simulink model "data_collection"  (R2024a)
settings: Solver=FixedStepAuto  StartTime=0.0  StopTime=inf  FixedStep=0.01  RelTol=1e-3
values from neighbouring files (symbols this model uses):
  omega_max = Simulink.Parameter(425.47)    [katech_automation.m]
  wind_type_toggle = 2    [katech_automation.m]    (also in katech_automation_HILS.m)
  window_size_ = Simulink.Parameter(100)    [katech_automation.m]    (also in katech_automation_HILS.m)
undefined symbols (not defined in the file or in its folder): rad, s, X, Y, Z
libraries: robotlib x28, simulink x14, aerolibconvert2 x2, sharedtransform x1, simulink_extras x1, eeGeneralControl x1
(part 2 of 2)

== matlab function data_collection/MATLAB Function11 ==
  data: wind_x_flag input; wind_y_flag input; u input; y output; toggle_swtich output
function [y, toggle_swtich] = fcn(wind_x_flag, wind_y_flag, u)
    coder.extrinsic('assignin'); % MATLAB 함수 사용을 알림


    % 이전 값을 저장할 persistent 변수 선언
    persistent prev_u;
    persistent toggle_state;
    persistent prev_flag;

    if isempty(prev_u)
        prev_u = -inf; % 초기 값 설정
    end

    if isempty(toggle_state)
        toggle_state = false; % 초기 토글 상태를 논리형으로 설정
    end

    if isempty(prev_flag)
        prev_flag    = false;
    end

    
    % 현재 플래그 레벨
    curr_flag = wind_x_flag || wind_y_flag;

    % 상승엣지 검출: 이전=0 & 현재=1
    if curr_flag && ~prev_flag
        toggle_state = ~toggle_state;
    end

    prev_flag = curr_flag;    % 엣지 검출을 위한 상태 갱신

    % 현재 토글 상태를 int32 형으로 변환하여 할당
    toggle_swtich = int32(toggle_state);
    % 현재 토글 상태를 출력
    % fprintf('toggle_state = %d \n', toggle_swtich);

    if toggle_state
        % 현재 값이 이전 값보다 큰지 확인
        if u > prev_u
            
            prev_u = u; % 이전 값을 현재 값으로 업데이트
            y = u; % 현재 값을 출력
        else
            y = prev_u; % 이전 값을 출력
        end
        assignin('base', 'max_z_error', y); % y 값을 MATLAB 기본 워크스페이스의 xy_error에 저장
    else
        % 토글 상태가 0일 때
        prev_u = 0;
        y = 0;
    end
end




    % if x_change || y_change
    % 
    %     % 현재 값이 이전 값보다 큰지 확인
    %     if u > prev_u
    %         assignin('base', 'xy_error', u);  % u 값을 MATLAB  워크스페이스(base는 MATLAB의 기본 워크스페이스를 의미)의 xy_error에 저장
    %         prev_u = u; % 이전 값을 현재 값으로 업데이트
    %         y = u; % 현재 값을 출력
    %     else
    %         y = prev_u; % 이전 값을 출력
    %     end
    % else
    %     assignin('base', 'xy_error', u);
    %     y = 0;
    % end

== matlab function data_collection/MATLAB Function12 ==
  data: endstep_xyz_error input; y output
function y = fcn(endstep_xyz_error)

% z_error 값을 기본 워크스페이스에 저장
assignin('base', 'endstep_xyz_error', endstep_xyz_error);

% 저장된 값을 반환
y = endstep_xyz_error;

end

== matlab function data_collection/MATLAB Function13 ==
  data: wind_toggle input; x_flag output; a1 input; a2 input; a3 input; a4 input; y_flag output
function [x_flag,y_flag] = fcn(wind_toggle,a1,a2,a3,a4)

% If wind_toggle is 
% 1 : Gust
% 2 : Normal Distribution
if wind_toggle == 1
    x_flag = a1;
    y_flag = a2;
else
    x_flag = a3;
    y_flag = a4;
end

end

== matlab function data_collection/MATLAB Function14 ==
  data: wind_x_flag input; wind_y_flag input; u input; y output; toggle_swtich output
function [y, toggle_swtich] = fcn(wind_x_flag, wind_y_flag, u)
    coder.extrinsic('assignin'); % MATLAB 함수 사용을 알림


    % 이전 값을 저장할 persistent 변수 선언
    persistent prev_u;
    persistent toggle_state;
    persistent prev_flag;

    if isempty(prev_u)
        prev_u = -inf; % 초기 값 설정
    end

    if isempty(toggle_state)
        toggle_state = false; % 초기 토글 상태를 논리형으로 설정
    end

    if isempty(prev_flag)
        prev_flag    = false;
    end

    
    % 현재 플래그 레벨
    curr_flag = wind_x_flag || wind_y_flag;

    % 상승엣지 검출: 이전=0 & 현재=1
    if curr_flag && ~prev_flag
        toggle_state = ~toggle_state;
    end

    prev_flag = curr_flag;    % 엣지 검출을 위한 상태 갱신

    % 현재 토글 상태를 int32 형으로 변환하여 할당
    toggle_swtich = int32(toggle_state);
    % 현재 토글 상태를 출력
    % fprintf('toggle_state = %d \n', toggle_swtich);

    if toggle_state
        % 현재 값이 이전 값보다 큰지 확인
        if u > prev_u
            
            prev_u = u; % 이전 값을 현재 값으로 업데이트
            y = u; % 현재 값을 출력
        else
            y = prev_u; % 이전 값을 출력
        end
        assignin('base', 'max_x_error', y); % y 값을 MATLAB 기본 워크스페이스의 xy_error에 저장
    else
        % 토글 상태가 0일 때
        prev_u = 0;
        y = 0;
    end
end




    % if x_change || y_change
    % 
    %     % 현재 값이 이전 값보다 큰지 확인
    %     if u > prev_u
    %         assignin('base', 'xy_error', u);  % u 값을 MATLAB  워크스페이스(base는 MATLAB의 기본 워크스페이스를 의미)의 xy_error에 저장
    %         prev_u = u; % 이전 값을 현재 값으로 업데이트
    %         y = u; % 현재 값을 출력
    %     else
    %         y = prev_u; % 이전 값을 출력
    %     end
    % else
    %     assignin('base', 'xy_error', u);
    %     y = 0;
    % end

== matlab function data_collection/Subsystem2/MATLAB Function5 ==
  data: wind_x_flag input; wind_y_flag input; u input; y output; toggle_swtich output
function [y, toggle_swtich] = fcn(wind_x_flag, wind_y_flag, u)
    coder.extrinsic('assignin'); % MATLAB 함수 사용을 알림


    % 이전 값을 저장할 persistent 변수 선언
    persistent prev_u;
    persistent toggle_state;
    persistent prev_flag;

    if isempty(prev_u)
        prev_u = -inf; % 초기 값 설정
    end

    if isempty(toggle_state)
        toggle_state = false; % 초기 토글 상태를 논리형으로 설정
    end

    if isempty(prev_flag)
        prev_flag    = false;
    end

    % 현재 플래그 레벨
    curr_flag = wind_x_flag || wind_y_flag;

    % 상승엣지 검출: 이전=0 & 현재=1
    if curr_flag && ~prev_flag
        toggle_state = ~toggle_state;
    end

    prev_flag = curr_flag;    % 엣지 검출을 위한 상태 갱신

    % 현재 토글 상태를 int32 형으로 변환하여 할당
    toggle_swtich = int32(toggle_state);
    % 현재 토글 상태를 출력
    % fprintf('toggle_state = %d \n', toggle_swtich);

    if toggle_state
        % 현재 값이 이전 값보다 큰지 확인
        if abs(u) > abs(prev_u)
            y = abs(prev_u); % 이전 값을 출력
            
        else
            prev_u = abs(u); % 이전 값을 현재 값으로 업데이트
            y = abs(u); % 현재 값을 출력
        end
        assignin('base', 'min_avg_array_FCM_saturated', y); % y 값을 MATLAB 기본 워크스페이스의 min_FCMW 저장
    else
        % 토글 상태가 0일 때
        prev_u = 1;
        y = 1;
    end
end




    % if x_change || y_change
    % 
    %     % 현재 값이 이전 값보다 큰지 확인
    %     if u > prev_u
    %         assignin('base', 'current_roll', u);  % u 값을 MATLAB  워크스페이스(base는 MATLAB의 기본 워크스페이스를 의미)의 current_roll에 저장
    %         prev_u = u; % 이전 값을 현재 값으로 업데이트
    %         y = u; % 현재 값을 출력
    %     else
    %         y = prev_u; % 이전 값을 출력
    %     end
    % else
    %     assignin('base', 'current_roll', u);
    %     y = 0;
    % end

== matlab function data_collection/MATLAB Function8 ==
  settings: updateMethod=DISCRETE
  data: xyz_error input; avg_array_xyz_error output; window_size_ parameter
function avg_array_xyz_error  = fcn(xyz_error, window_size_)

coder.extrinsic('calculate_xyzerror.m');

% persistent 변수 선언
persistent initialized avg_array_xyz_error_;

% 초기화가 필요할 때만 실행
if isempty(initialized)
    initialized = true; % 초기화 완료 표시
    one_or_zero = 0;
    one_or_zero_ = 0;
    avg_array_xyz_error = 0.0;
    avg_array_xyz_error_ = 0.0;

    disp('initialized. in MATLAB Function8');
    % disp('window_size_ in MATLAB Function8'); disp(window_size_);
end


[one_or_zero_, avg_array_xyz_error_] = calculate_xyzerror(xyz_error,window_size_);

one_or_zero = one_or_zero_;
avg_array_xyz_error = avg_array_xyz_error_;





end

== matlab function data_collection/MATLAB Function15 ==
  data: wind_x_flag input; wind_y_flag input; u input; y output; toggle_swtich output
function [y, toggle_swtich] = fcn(wind_x_flag, wind_y_flag, u)
    coder.extrinsic('assignin'); % MATLAB 함수 사용을 알림


    % 이전 값을 저장할 persistent 변수 선언
    persistent prev_u;
    persistent toggle_state;
    persistent prev_flag;

    if isempty(prev_u)
        prev_u = -inf; % 초기 값 설정
    end

    if isempty(toggle_state)
        toggle_state = false; % 초기 토글 상태를 논리형으로 설정
    end

    if isempty(prev_flag)
        prev_flag    = false;
    end

    
    % 현재 플래그 레벨
    curr_flag = wind_x_flag || wind_y_flag;

    % 상승엣지 검출: 이전=0 & 현재=1
    if curr_flag && ~prev_flag
        toggle_state = ~toggle_state;
    end

    prev_flag = curr_flag;    % 엣지 검출을 위한 상태 갱신

    % 현재 토글 상태를 int32 형으로 변환하여 할당
    toggle_swtich = int32(toggle_state);
    % 현재 토글 상태를 출력
    % fprintf('toggle_state = %d \n', toggle_swtich);

    if toggle_state
        % 현재 값이 이전 값보다 큰지 확인
        if u > prev_u
            
            prev_u = u; % 이전 값을 현재 값으로 업데이트
            y = u; % 현재 값을 출력
        else
            y = prev_u; % 이전 값을 출력
        end
        assignin('base', 'max_avg_xyz_error', y); % y 값을 MATLAB 기본 워크스페이스의 max_avg_xyz_error 에 저장
    else
        % 토글 상태가 0일 때
        prev_u = 0;
        y = 0;
    end
end




    % if x_change || y_change
    % 
    %     % 현재 값이 이전 값보다 큰지 확인
    %     if u > prev_u
    %         assignin('base', 'xy_error', u);  % u 값을 MATLAB  워크스페이스(base는 MATLAB의 기본 워크스페이스를 의미)의 xy_error에 저장
    %         prev_u = u; % 이전 값을 현재 값으로 업데이트
    %         y = u; % 현재 값을 출력
    %     else
    %         y = prev_u; % 이전 값을 출력
    %     end
    % else
    %     assignin('base', 'xy_error', u);
    %     y = 0;
    % end

== matlab function data_collection/MATLAB Function16 ==
  data: u input
function write_pos_err(u)
    assignin('base', 'position_error', u);
end

== matlab function data_collection/Subsystem2/MATLAB Function7 ==
  data: u input
function write_fcmw(u)
    assignin('base', 'FCMW_saturated', u);
end

== matlab function data_collection/MATLAB Function1 ==
  data: wind_x_flag input; wind_y_flag input; u input; y output; toggle_swtich output
function [y, toggle_swtich] = fcn(wind_x_flag, wind_y_flag, u)
    coder.extrinsic('assignin'); % MATLAB 함수 사용을 알림


    % 이전 값을 저장할 persistent 변수 선언
    persistent prev_u;
    persistent toggle_state;
    persistent prev_flag;

    if isempty(prev_u)
        prev_u = -inf; % 초기 값 설정
    end

    if isempty(toggle_state)
        toggle_state = false; % 초기 토글 상태를 논리형으로 설정
    end

    if isempty(prev_flag)
        prev_flag    = false;
    end

    
    % 현재 플래그 레벨
    curr_flag = wind_x_flag || wind_y_flag;

    % 상승엣지 검출: 이전=0 & 현재=1
    if curr_flag && ~prev_flag
        toggle_state = ~toggle_state;
    end

    prev_flag = curr_flag;    % 엣지 검출을 위한 상태 갱신

    % 현재 토글 상태를 int32 형으로 변환하여 할당
    toggle_swtich = int32(toggle_state);
    % 현재 토글 상태를 출력
    % fprintf('toggle_state = %d \n', toggle_swtich);

    if toggle_state
        % 현재 값이 이전 값보다 큰지 확인
        if abs(u) > abs(prev_u)
            
            prev_u = u; % 이전 값을 현재 값으로 업데이트
            y = u; % 현재 값을 출력
        else
            y = prev_u; % 이전 값을 출력
        end
        assignin('base', 'max_roll', y); % y 값을 MATLAB 기본 워크스페이스의 xy_error에 저장
    else
        % 토글 상태가 0일 때
        prev_u = 0;
        y = 0;
    end
end




    % if x_change || y_change
    % 
    %     % 현재 값이 이전 값보다 큰지 확인
    %     if u > prev_u
    %         assignin('base', 'xy_error', u);  % u 값을 MATLAB  워크스페이스(base는 MATLAB의 기본 워크스페이스를 의미)의 xy_error에 저장
    %         prev_u = u; % 이전 값을 현재 값으로 업데이트
    %         y = u; % 현재 값을 출력
    %     else
    %         y = prev_u; % 이전 값을 출력
    %     end
    % else
    %     assignin('base', 'xy_error', u);
    %     y = 0;
    % end

== matlab function data_collection/MATLAB Function ==
  data: wind_x_flag input; wind_y_flag input; u input; y output; toggle_swtich output
function [y, toggle_swtich] = fcn(wind_x_flag, wind_y_flag, u)
    coder.extrinsic('assignin'); % MATLAB 함수 사용을 알림


    % 이전 값을 저장할 persistent 변수 선언
    persistent prev_u;
    persistent toggle_state;
    persistent prev_flag;

    if isempty(prev_u)
        prev_u = -inf; % 초기 값 설정
    end

    if isempty(toggle_state)
        toggle_state = false; % 초기 토글 상태를 논리형으로 설정
    end

    if isempty(prev_flag)
        prev_flag    = false;
    end

    
    % 현재 플래그 레벨
    curr_flag = wind_x_flag || wind_y_flag;

    % 상승엣지 검출: 이전=0 & 현재=1
    if curr_flag && ~prev_flag
        toggle_state = ~toggle_state;
    end

    prev_flag = curr_flag;    % 엣지 검출을 위한 상태 갱신

    % 현재 토글 상태를 int32 형으로 변환하여 할당
    toggle_swtich = int32(toggle_state);
    % 현재 토글 상태를 출력
    % fprintf('toggle_state = %d \n', toggle_swtich);

    if toggle_state
        % 현재 값이 이전 값보다 큰지 확인
        if u > prev_u
            
            prev_u = u; % 이전 값을 현재 값으로 업데이트
            y = u; % 현재 값을 출력
        else
            y = prev_u; % 이전 값을 출력
        end
        assignin('base', 'max_xy_error', y); % y 값을 MATLAB 기본 워크스페이스의 xy_error에 저장
    else
        % 토글 상태가 0일 때
        prev_u = 0;
        y = 0;
    end
end




    % if x_change || y_change
    % 
    %     % 현재 값이 이전 값보다 큰지 확인
    %     if u > prev_u
    %         assignin('base', 'xy_error', u);  % u 값을 MATLAB  워크스페이스(base는 MATLAB의 기본 워크스페이스를 의미)의 xy_error에 저장
    %         prev_u = u; % 이전 값을 현재 값으로 업데이트
    %         y = u; % 현재 값을 출력
    %     else
    %         y = prev_u; % 이전 값을 출력
    %     end
    % else
    %     assignin('base', 'xy_error', u);
    %     y = 0;
    % end

== matlab function data_collection/MATLAB Function2 ==
  data: endstep_z_error input; y output
function y = fcn(endstep_z_error)

% z_error 값을 기본 워크스페이스에 저장
assignin('base', 'endstep_z_error', endstep_z_error);

% 저장된 값을 반환
y = endstep_z_error;

end

== matlab function data_collection/MATLAB Function3 ==
  data: endstep_y_error input; y output
function y = fcn(endstep_y_error)

% z_error 값을 기본 워크스페이스에 저장
assignin('base', 'endstep_y_error', endstep_y_error);

% 저장된 값을 반환
y = endstep_y_error;

end

== matlab function data_collection/MATLAB Function4 ==
  data: endstep_x_error input; y output
function y = fcn(endstep_x_error)

% z_error 값을 기본 워크스페이스에 저장
assignin('base', 'endstep_x_error', endstep_x_error);

% 저장된 값을 반환
y = endstep_x_error;

end

== matlab function data_collection/MATLAB Function5 ==
  data: xy_error input; y output
function y = two_norm(xy_error)
    coder.extrinsic('norm'); % MATLAB 함수 사용을 알림
    
    

    
    % 'y'를 명확히 초기화
    y = 0; 
    
y = norm(xy_error,2);

== matlab function data_collection/MATLAB Function6 ==
  data: wind_x_flag input; wind_y_flag input; u input; y output; toggle_swtich output
function [y, toggle_swtich] = fcn(wind_x_flag, wind_y_flag, u)
    coder.extrinsic('assignin'); % MATLAB 함수 사용을 알림


    % 이전 값을 저장할 persistent 변수 선언
    persistent prev_u;
    persistent toggle_state;
    persistent prev_flag;

    if isempty(prev_u)
        prev_u = -inf; % 초기 값 설정
    end

    if isempty(toggle_state)
        toggle_state = false; % 초기 토글 상태를 논리형으로 설정
    end

    if isempty(prev_flag)
        prev_flag    = false;
    end

    
    % 현재 플래그 레벨
    curr_flag = wind_x_flag || wind_y_flag;

    % 상승엣지 검출: 이전=0 & 현재=1
    if curr_flag && ~prev_flag
        toggle_state = ~toggle_state;
    end

    prev_flag = curr_flag;    % 엣지 검출을 위한 상태 갱신

    % 현재 토글 상태를 int32 형으로 변환하여 할당
    toggle_swtich = int32(toggle_state);
    % 현재 토글 상태를 출력
    % fprintf('toggle_state = %d \n', toggle_swtich);

    if toggle_state
        % 현재 값이 이전 값보다 큰지 확인
        if u > prev_u
            
            prev_u = u; % 이전 값을 현재 값으로 업데이트
            y = u; % 현재 값을 출력
        else
            y = prev_u; % 이전 값을 출력
        end
        assignin('base', 'max_y_error', y); % y 값을 MATLAB 기본 워크스페이스의 xy_error에 저장
    else
        % 토글 상태가 0일 때
        prev_u = 0;
        y = 0;
    end
end




    % if x_change || y_change
    % 
    %     % 현재 값이 이전 값보다 큰지 확인
    %     if u > prev_u
    %         assignin('base', 'xy_error', u);  % u 값을 MATLAB  워크스페이스(base는 MATLAB의 기본 워크스페이스를 의미)의 xy_error에 저장
    %         prev_u = u; % 이전 값을 현재 값으로 업데이트
    %         y = u; % 현재 값을 출력
    %     else
    %         y = prev_u; % 이전 값을 출력
    %     end
    % else
    %     assignin('base', 'xy_error', u);
    %     y = 0;
    % end

== matlab function data_collection/MATLAB Function7 ==
  data: wind_x_flag input; wind_y_flag input; u input; y output; toggle_swtich output
function [y, toggle_swtich] = fcn(wind_x_flag, wind_y_flag, u)
    coder.extrinsic('assignin'); % MATLAB 함수 사용을 알림


    % 이전 값을 저장할 persistent 변수 선언
    persistent prev_u;
    persistent toggle_state;
    persistent prev_flag;

    if isempty(prev_u)
        prev_u = -inf; % 초기 값 설정
    end

    if isempty(toggle_state)
        toggle_state = false; % 초기 토글 상태를 논리형으로 설정
    end

    if isempty(prev_flag)
        prev_flag    = false;
    end

    
    % 현재 플래그 레벨
    curr_flag = wind_x_flag || wind_y_flag;

    % 상승엣지 검출: 이전=0 & 현재=1
    if curr_flag && ~prev_flag
        toggle_state = ~toggle_state;
    end

    prev_flag = curr_flag;    % 엣지 검출을 위한 상태 갱신

    % 현재 토글 상태를 int32 형으로 변환하여 할당
    toggle_swtich = int32(toggle_state);
    % 현재 토글 상태를 출력
    % fprintf('toggle_state = %d \n', toggle_swtich);

    if toggle_state
        % 현재 값이 이전 값보다 큰지 확인
        if u > prev_u
            
            prev_u = u; % 이전 값을 현재 값으로 업데이트
            y = u; % 현재 값을 출력
        else
            y = prev_u; % 이전 값을 출력
        end
        assignin('base', 'max_xyz_error', y); % y 값을 MATLAB 기본 워크스페이스의 xy_error에 저장
    else
        % 토글 상태가 0일 때
        prev_u = 0;
        y = 0;
    end
end




    % if x_change || y_change
    % 
    %     % 현재 값이 이전 값보다 큰지 확인
    %     if u > prev_u
    %         assignin('base', 'xy_error', u);  % u 값을 MATLAB  워크스페이스(base는 MATLAB의 기본 워크스페이스를 의미)의 xy_error에 저장
    %         prev_u = u; % 이전 값을 현재 값으로 업데이트
    %         y = u; % 현재 값을 출력
    %     else
    %         y = prev_u; % 이전 값을 출력
    %     end
    % else
    %     assignin('base', 'xy_error', u);
    %     y = 0;
    % end
